simulink model "dcIntrocomplete"  (Simulink 10.1)
settings: Solver=ode45  StartTime=0.0  StopTime=10.0  RelTol=1e-3  EnableMultiTasking=on
PreLoadFcn:
  | % Motor Parameters
  | 
  | J=0.01;     %kg*m^2
  | b=0.1;      %N*m/(rad/s)
  | K=0.01;     %V/(rad/s)
  | R=1;        %Ohm
  | L=0.5;      %H
undefined symbols (not defined in the file): Kd, Ki, Kp, wb, wh
libraries: fod x2
settings Model: Creator=deastman  LastModifiedBy=Aman Saxena
settings DataIOCC: LimitDataPoints=on  SignalLoggingSaveFormat=ModelDataLogs
settings OptimizationCC: ExpressionDepthLimit=2147483647  InitFltsAndDblsToZero=on
settings DebuggingCC: SolverPrmCheckMsg=warning  FcnCallInpInsideContextMsg=warning  StateNameClashWarn=warning

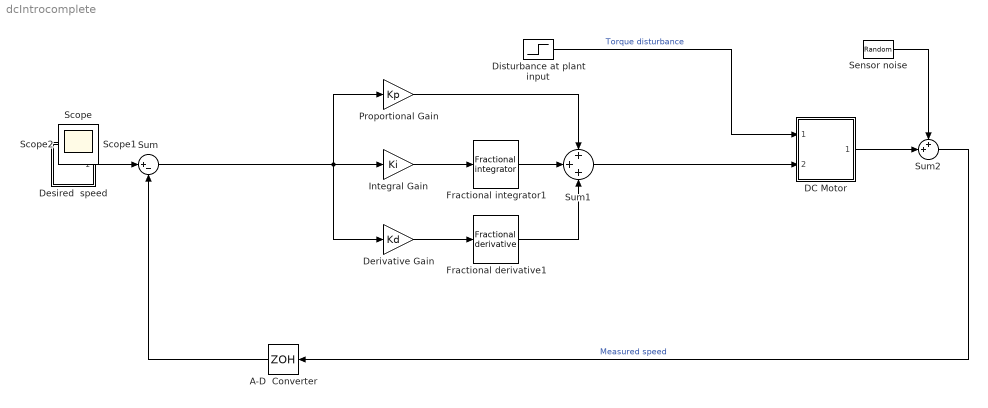
== system dcIntrocomplete ==
  " Disturbance at plant input" : Step  Time=5  After=0.2  SampleTime=0
  A-D  Converter : ZeroOrderHold  SampleTime=0.02
  DC Motor : Subsystem  mask(DC Motor){b=b, J=J, K=K, R=R, L=L}
      mask prompts: b "Damping:"; J "Inertia:"; K "Back EMF:"; R "Resistance:"; L "Inductance:"
      mask help: An ideal model of a DC Motor
      mask Help: This is <b>more elaborate<b> help.
      mask Display: image(imread('dcmotor.jpg'))
  Derivative Gain : Gain  Gain=Kd
  Desired  speed : Subsystem
  Fractional derivative1 : fod/Fractional derivative  gam=mic  ww=[wb; wh]  n=N  nFod=off
      settings: SourceProductName=FOMCON Toolbox
  Fractional integrator1 : fod/Fractional integrator  gam=lambda  ww=[wb; wh]  n=N  nFod=off
      settings: SourceProductName=FOMCON Toolbox
  Integral Gain : Gain  Gain=Ki
  Proportional Gain : Gain  Gain=Kp
  Sensor noise : RandomNumber  Variance=0.05  SampleTime=0
  Sum : Sum  Inputs=|+-
  Sum1 : Sum  Inputs=+++  InputSameDT=on  SaturateOnIntegerOverflow=on  OutDataTypeStr=Inherit: Same as first input
  Sum2 : Sum  Inputs=++|
  Scope : Scope
  Scope1 : Scope
  Scope2 : Scope
  wires:
  " Disturbance at plant input"/1 -> DC Motor/1(Torque)  "Torque disturbance"
  Desired  speed/1(Speed) -> Sum/1
  DC Motor/1(Speed) -> Sum2/2
  Sum2/1 -> A-D  Converter/1  "Measured speed"
  Sensor noise/1 -> Sum2/1
  A-D  Converter/1 -> Sum/2
  Integral Gain/1 -> Fractional integrator1/1
  Fractional derivative1/1 -> Sum1/3
  Derivative Gain/1 -> Fractional derivative1/1
  Sum/1 -> Proportional Gain/1, Derivative Gain/1, Integral Gain/1
  Fractional integrator1/1 -> Sum1/2
  Proportional Gain/1 -> Sum1/1
  Sum1/1 -> DC Motor/2(Voltage)

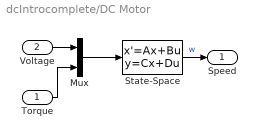
== system dcIntrocomplete/DC Motor ==
  Torque : Inport
  Voltage : Inport  Port=2
  Mux : Mux  Inputs=2
  State-Space : StateSpace  A=[-b/J K/J; -K/L -R/L]  B=[0 -1/J; 1/L 0]  C=[1 0]  D=[0 0]  InitialCondition=0
  Speed : Outport
  wires:
  Mux/1 -> State-Space/1
  Voltage/1 -> Mux/1
  State-Space/1 -> Speed/1  "w"
  Torque/1 -> Mux/2

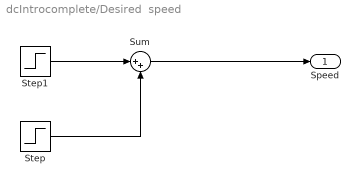
== system dcIntrocomplete/Desired  speed ==
  Step : Step  Time=7  After=-4  SampleTime=0.02
  Step1 : Step  After=2  SampleTime=0.02
  Sum : Sum  Inputs=|++
  Speed : Outport
  wires:
  Step/1 -> Sum/2
  Step1/1 -> Sum/1
  Sum/1 -> Speed/1
